simulink model "multiAgents5_2"  (Simulink 7.0)
settings: Solver=ode23tb  StartTime=0.0  StopTime=50  RelTol=1e-3
values from neighbouring files (symbols this model uses):
  A1 = toMatrix(block.InputPort(1).Data)    [assignmentDynamics.m]    (also in initMultiAgents.m = makeIncludedAngleMatrix(zeta))
  A2 = toMatrix(block.InputPort(2).Data)    [assignmentDynamics.m]    (also in initMultiAgents.m = makeIncludedAngleMatrix(tmp))
  D = kron(eye(6),Di)    [initMultiAgents.m]
settings Model: Creator=wizest  LastModifiedBy=wizest

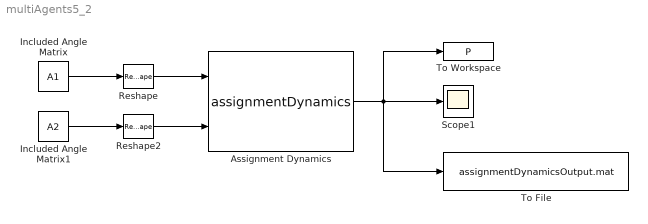
== system multiAgents5_2 ==
  Assignment Dynamics : M-S-Function  FunctionName=assignmentDynamics
  Included Angle Matrix : Constant  Value=A1  OutDataType=sfix(16)  OutScaling=2^0
  Included Angle Matrix1 : Constant  Value=A2  OutDataType=sfix(16)  OutScaling=2^0
  Reshape : Reshape  OutputDimensionality=Column vector (2-D)
  Reshape2 : Reshape  OutputDimensionality=Column vector (2-D)
  Scope1 : Scope
      settings: TimeRange=5  YMin=-0.5  YMax=1.1
  To File : ToFile  Filename=assignmentDynamicsOutput.mat
  To Workspace : ToWorkspace  VariableName=P  SampleTime=-1  SaveFormat=Structure
  wires:
  Assignment Dynamics/1 -> Scope1/1, To Workspace/1, To File/1
  Reshape/1 -> Assignment Dynamics/1
  Included Angle Matrix/1 -> Reshape/1
  Included Angle Matrix1/1 -> Reshape2/1
  Reshape2/1 -> Assignment Dynamics/2
